simulink subsystem "GCI_to_ECEF"  (R2022a)
settings: Solver=VariableStepAuto  StartTime=0.0  StopTime=10.0  RelTol=1e-3
libraries: simulink_extras x1
settings Model: Creator=samuel  LastModifiedBy=samuel

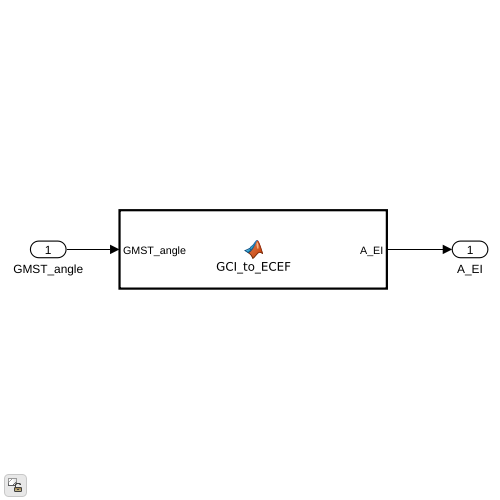
[thumbnail: Simulink's stored preview of the top-level diagram]
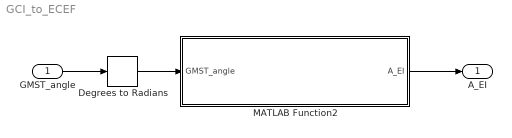
== system GCI_to_ECEF ==
  GMST_angle : Inport
  Degrees to Radians : simulink_extras/Transformations/Degrees to Radians
  MATLAB Function2 : MATLAB Function  TreatAsAtomicUnit=on
  A_EI : Outport
  wires:
  MATLAB Function2/1(A_EI) -> A_EI/1
  Degrees to Radians/1 -> MATLAB Function2/1(GMST_angle)
  GMST_angle/1 -> Degrees to Radians/1

== matlab function GCI_to_ECEF/MATLAB Function2 ==
  data: GMST_angle input; A_EI output
function A_EI = GCI_to_ECEF(GMST_angle)

    A_EI = [cos(GMST_angle) sin(GMST_angle) 0 ;
            -sin(GMST_angle) cos(GMST_angle) 0 ;
            0 0 1];
